simulink model "tanks"  (R2025b)
settings: Solver=VariableStepAuto  StartTime=0.0  StopTime=10.0  RelTol=1e-3
model workspace (MAT data in the model file):
  sine_amp = 0.2
values from neighbouring files (symbols this model uses):
  a = 0.2    [tanks.m]
  omega = u(3)    [pendulum_func.m]    (also in tanks.m = 5)
  qbar = 1.5    [tanks.m]
settings Model: Creator=jbrouill  LastModifiedBy=seby
settings SolverCC: AlgebraicLoopSolver=TrustRegion
settings DataIOCC: Refine=10
settings DebuggingCC: UnconnectedInputMsg=warning  UnconnectedOutputMsg=warning  UnconnectedLineMsg=warning
settings ModelReferenceCC: EnableRefExpFcnMdlSchedulingChecks=on
settings RTWCC: GPUComputeCapability=3.5

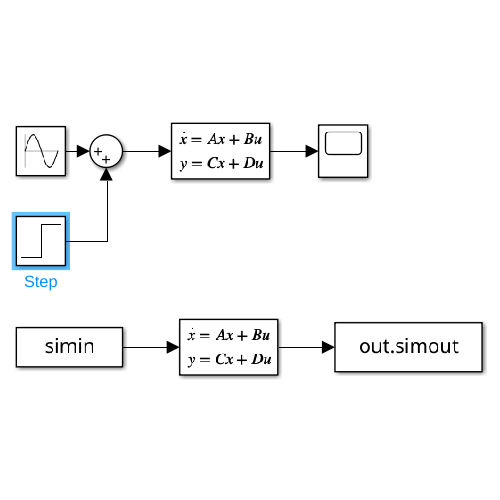
[thumbnail: Simulink's stored preview of the top-level diagram]
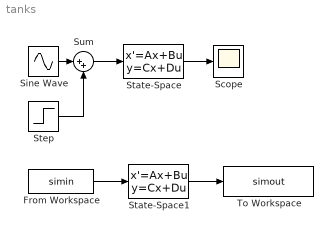
== system tanks ==
  From Workspace : FromWorkspace  VariableName=simin
  Scope : Scope
      settings: ActiveDisplayYMinimum=0.33860647335424521  ActiveDisplayYMaximum=1.7099487195306404
  Sine Wave : Sin  Amplitude=a  Frequency=omega  SampleTime=0
  State-Space : StateSpace  A=[-3 0; 3 -5]  B=[1 ; 0]  C=[0 5]  D=[0]  InitialCondition=[0.1 ; 0.1]
  State-Space1 : StateSpace  A=[-3 0; 3 -5]  B=[1 ; 0]  C=[0 5]  D=[0]  InitialCondition=[0.1 ; 0.1]
  Step : Step  Time=0  After=qbar  SampleTime=0
  Sum : Sum  Inputs=|++
  To Workspace : ToWorkspace  VariableName=simout  SaveFormat=Timeseries  SampleTime=-1
  wires:
  Step/1 -> Sum/2
  State-Space/1 -> Scope/1
  Sum/1 -> State-Space/1
  Sine Wave/1 -> Sum/1
  State-Space1/1 -> To Workspace/1
  From Workspace/1 -> State-Space1/1
